simulink model "GTO_characteristics"  (R2020a)
settings: Solver=VariableStepAuto  StartTime=0.0  StopTime=0.1  RelTol=1e-3
libraries: powerlib x4, simulink x1
settings Model: Creator=Naeem Mohammad  LastModifiedBy=Naeem Mohammad

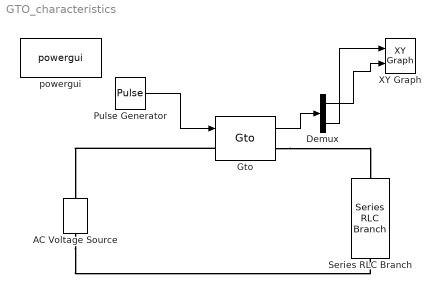
== system GTO_characteristics ==
  AC Voltage Source : powerlib/Electrical Sources/AC Voltage Source  Amplitude=12  Phase=0  Frequency=60  SampleTime=0  Measurements=None  BusType=swing  Pref=10e3  Qref=0  Qmin=-inf  Qmax=+inf
  Demux : Demux  Outputs=2
  Gto : powerlib/Power Electronics/Gto  Ron=0.001  Lon=0  Vf=1  Tf=10e-6  Tt=20e-6  IC=0  Rs=1e5  Cs=inf  Measurements=on
      settings: SourceProductBaseCode=PS
  Pulse Generator : DiscretePulseGenerator  PulseType=Time based  Period=0.0167  PulseWidth=70
  Series RLC Branch : powerlib/Elements/Series RLC Branch  LConnTagsString=__new0  RConnTagsString=__new0  BranchType=R  Resistance=10  Inductance=1e-3  SetiL0=off  InitialCurrent=0  Capacitance=1e-6  Setx0=off  InitialVoltage=0  Measurements=None
  XY Graph : simulink/Sinks/XY Graph  xmin=-3  xmax=3  ymin=-3  ymax=3  st=-1
  powergui : powerlib/powergui  Priority=1  SimulationMode=Discrete  SampleTime=50e-6  frequency=60  Iterations=50  frequencyindice=0  Pbase=100e6  ErrMax=1e-4  UnitsV=kV  UnitsW=MW  buscounter=0  FunctionMessages=off  echomessages=off  EnableUseOfTLC=off  CurrentSourceSwitches=off  DisableSnubberDevices=off  DisableRonSwitches=off  DisableVfSwitches=off  DisplayEquations=off  AutomaticDiscreteSolvers=off  SolverType=Tustin/Backward Euler (TBE)  Interpol=off  ExternalGateDelay=off  methode=off  Ts=100  x0status=blocks  SPID=on  SwTol=0  HookPort=off  NonlinearTolerance=1e-4  nMaxIteration=100  ContinueOnMaxIteration=off  RestoreLinks=warning  ResistiveCurrentMeasurement=off  Frange=[0:2:500]  Ylog=off  Xlog=on  ShowGrid=off  save=off  variable=ZData  structure=0  ZoomFFT=off  StartTime=0.0  cycles=1  DisplayStyle=1  fundamental=60  FreqAxis=off  MaxFrequency=1000  frequencyindicesteady=1  RmsSteady=1  display=off
  wires:
  Pulse Generator/1 -> Gto/1
  Gto/1 -> Demux/1
  Demux/1 -> XY Graph/2
  Demux/2 -> XY Graph/1
  connections:
  Gto/RConn1 -- Series RLC Branch/RConn1
  Gto/LConn1 -- AC Voltage Source/RConn1
  AC Voltage Source/LConn1 -- Series RLC Branch/LConn1
